simulink model "control_feedback_and_plant"  (R2023b)
settings: Solver=FixedStepAuto  StartTime=0.0  StopTime=500  FixedStep=0.01  RelTol=1e-3
settings Model: Creator=bhargavjha  LastModifiedBy=bhargavjha

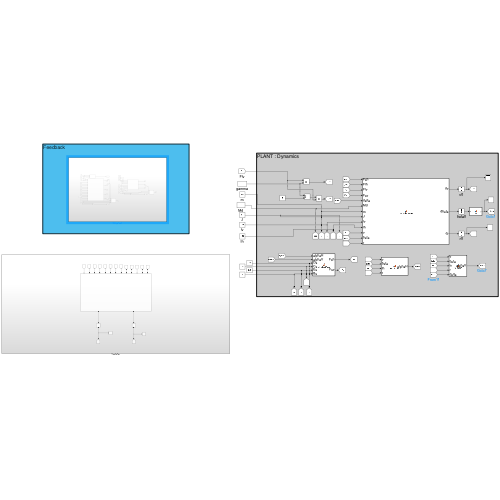
[thumbnail: Simulink's stored preview of the top-level diagram]
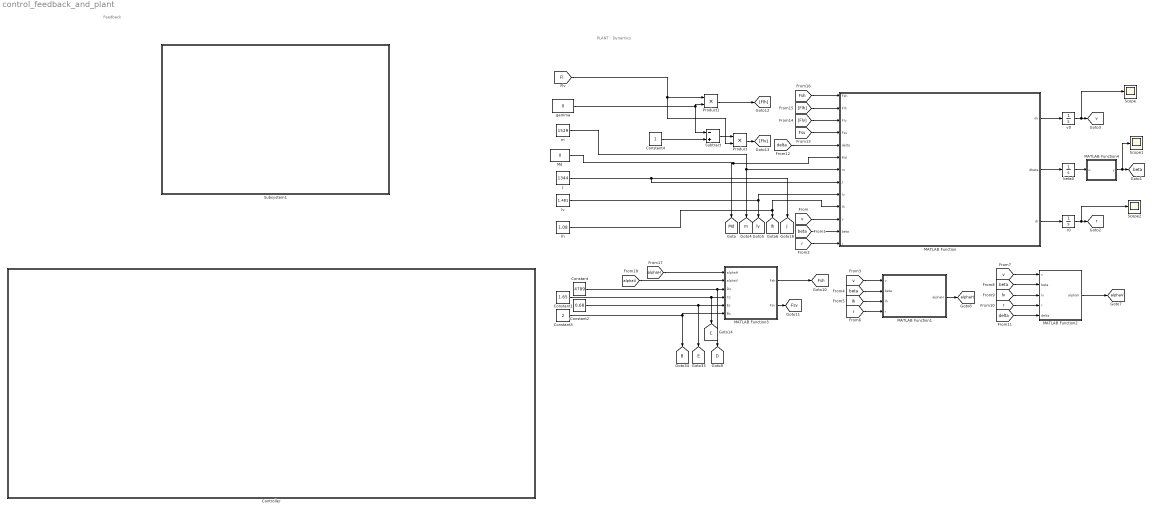
== system control_feedback_and_plant ==
  note: PLANT : Dynamics
  note: Feedback
  Constant : Constant  Value=4789
  Constant1 : Constant  Value=1.65
  Constant2 : Constant  Value=0.68
  Constant3 : Constant  Value=2
  Constant4 : Constant
  Controller : Subsystem
  J : Constant  Value=1344
  MATLAB Function : MATLAB Function  TreatAsAtomicUnit=on
  MATLAB Function1 : MATLAB Function  TreatAsAtomicUnit=on
  MATLAB Function2 : MATLAB Function  TreatAsAtomicUnit=on
  MATLAB Function3 : MATLAB Function  TreatAsAtomicUnit=on
  MATLAB Function4 : MATLAB Function  TreatAsAtomicUnit=on
  Md : Constant  Value=0
  Product : Product
  Product1 : Product
  Scope : Scope
  Scope1 : Scope
  Scope2 : Scope
  Subsystem1 : Subsystem
  Subtract : Sum  Inputs=-+
  beta0 : Integrator  InitialCondition=0.9
  gamma : Constant  Value=0
  lh : Constant  Value=1.08
  lv : Constant  Value=1.481
  m : Constant  Value=1529
  r0 : Integrator  InitialCondition=0.1
  v0 : Integrator  InitialCondition=0.1
  tag scope: B=global, C=global, D=global, E=global, Fsh=global, Fsv=global, J=global, Md=global, alphaH=global, alphaV=global, beta=global, lh=global, lv=global, m=global, r=global, v=global
  wires:
  [lv] -> MATLAB Function2/3(lv)
  MATLAB Function1/1(alphaH) -> [alphaH]
  MATLAB Function3/2(Fsv) -> [Fsv]
  v0/1 -> Scope/1, [v]
  lh/1 -> MATLAB Function/10(lh), [lh]
  MATLAB Function/1(dv) -> v0/1
  [beta] -> MATLAB Function1/2(beta)
  [v] -> MATLAB Function/11(v)
  J/1 -> [J], MATLAB Function/8(J)
  [Flh] -> MATLAB Function/2(Flh)
  Subtract/1 -> Product/1
  [Fsh] -> MATLAB Function/1(Fsh)
  m/1 -> [m], MATLAB Function/7(m)
  [v] -> MATLAB Function2/1(v)
  Product/1 -> [Flv]
  [r] -> MATLAB Function2/4(r)
  [v] -> MATLAB Function1/1(v)
  Constant3/1 -> MATLAB Function3/6(Bs), [B]
  gamma/1 -> Product1/2, Subtract/1
  lv/1 -> MATLAB Function/9(lv), [lv]
  [lh] -> MATLAB Function1/3(lh)
  MATLAB Function2/1(alphaV) -> [alphaV]
  Constant/1 -> [D], MATLAB Function3/3(Ds)
  Constant1/1 -> [C], MATLAB Function3/4(Cs)
  [beta] -> MATLAB Function/12(beta)
  Constant4/1 -> Subtract/2
  [delta] -> MATLAB Function/5(delta)
  Constant2/1 -> [E], MATLAB Function3/5(Es)
  MATLAB Function/3(dr) -> r0/1
  [alphaH] -> MATLAB Function3/1(alphaH)
  [Flv] -> MATLAB Function/3(Flv)
  [r] -> MATLAB Function/13(r)
  beta0/1 -> MATLAB Function4/1(u)
  MATLAB Function/2(dbeta) -> beta0/1
  [beta] -> MATLAB Function2/2(beta)
  Product1/1 -> [Flh]
  r0/1 -> Scope2/1, [r]
  [delta] -> MATLAB Function2/5(delta)
  [r] -> MATLAB Function1/4(r)
  MATLAB Function3/1(Fsh) -> [Fsh]
  Md/1 -> [Md], MATLAB Function/6(Md)
  [alphaV] -> MATLAB Function3/2(alphaV)
  [Fsv] -> MATLAB Function/4(Fsv)
  [Fl] -> Product/2, Product1/1
  MATLAB Function4/1(y) -> Scope1/1, [beta]

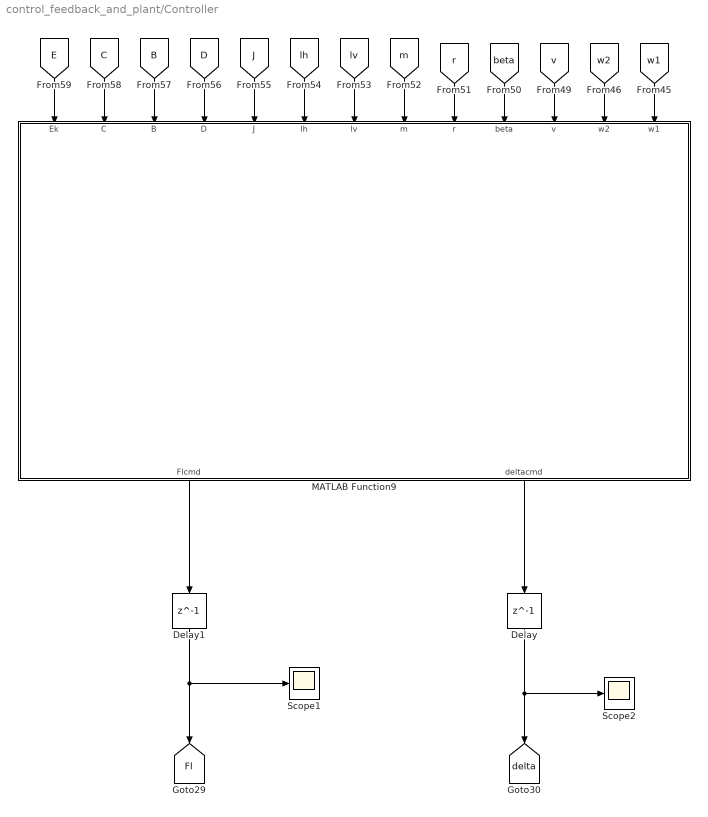
== system control_feedback_and_plant/Controller ==
  Delay : Delay  DelayLength=1
  Delay1 : Delay  DelayLength=1
  MATLAB Function9 : MATLAB Function  TreatAsAtomicUnit=on
  Scope1 : Scope
  Scope2 : Scope
  tag scope: Fl=global, delta=global
  wires:
  [B] -> MATLAB Function9/3(B)
  [C] -> MATLAB Function9/2(C)
  [E] -> MATLAB Function9/1(Ek)
  [lh] -> MATLAB Function9/6(lh)
  [w2] -> MATLAB Function9/12(w2)
  [m] -> MATLAB Function9/8(m)
  [beta] -> MATLAB Function9/10(beta)
  [w1] -> MATLAB Function9/13(w1)
  [D] -> MATLAB Function9/4(D)
  [J] -> MATLAB Function9/5(J)
  [r] -> MATLAB Function9/9(r)
  [lv] -> MATLAB Function9/7(lv)
  [v] -> MATLAB Function9/11(v)
  MATLAB Function9/2(deltacmd) -> Delay/1
  Delay/1 -> Scope2/1, [delta]
  Delay1/1 -> [Fl], Scope1/1
  MATLAB Function9/1(Flcmd) -> Delay1/1

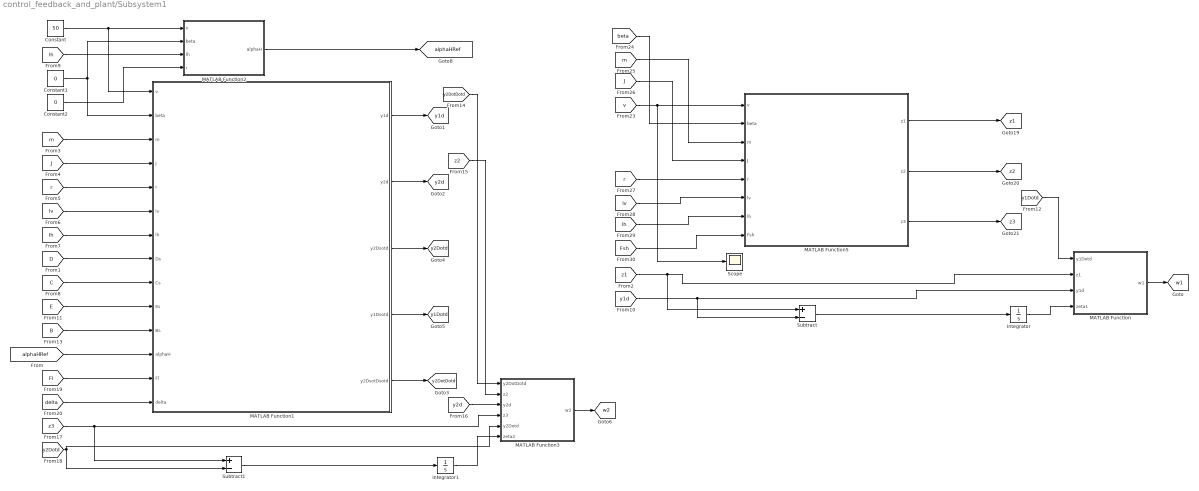
== system control_feedback_and_plant/Subsystem1 ==
  Constant : Constant  Value=50
  Constant1 : Constant  Value=0
  Constant2 : Constant  Value=0
  Integrator : Integrator
  Integrator1 : Integrator
  MATLAB Function : MATLAB Function  TreatAsAtomicUnit=on
  MATLAB Function1 : MATLAB Function  TreatAsAtomicUnit=on
  MATLAB Function2 : MATLAB Function  TreatAsAtomicUnit=on
  MATLAB Function3 : MATLAB Function  TreatAsAtomicUnit=on
  MATLAB Function5 : MATLAB Function  TreatAsAtomicUnit=on
  Scope : Scope
  Subtract : Sum  Inputs=+-
  Subtract1 : Sum  Inputs=+-
  tag scope: alphaHRef=global, w1=global, w2=global, y1Dotd=global, y1d=global, y2DotDotd=global, y2Dotd=global, y2d=global, z1=global, z2=global, z3=global
  wires:
  MATLAB Function3/1(w2) -> [w2]
  Integrator1/1 -> MATLAB Function3/6(zeta2)
  [y2d] -> MATLAB Function3/3(y2d)
  Integrator/1 -> MATLAB Function/4(zeta1)
  [y2DotDotd] -> MATLAB Function3/1(y2DotDotd)
  Subtract/1 -> Integrator/1
  Subtract1/1 -> Integrator1/1
  MATLAB Function1/5(y2DsotDsotd) -> [y2DotDotd]
  MATLAB Function1/4(y1Dsotd) -> [y1Dotd]
  MATLAB Function1/3(y2Dsotd) -> [y2Dotd]
  MATLAB Function1/2(y2d) -> [y2d]
  MATLAB Function2/1(alphaH) -> [alphaHRef]
  [z1] -> Subtract/1, MATLAB Function/2(z1)
  [Fsh] -> MATLAB Function5/8(Fsh)
  [lh] -> MATLAB Function5/7(lh)
  MATLAB Function/1(w1) -> [w1]
  [y1d] -> Subtract/2, MATLAB Function/3(y1d)
  [lv] -> MATLAB Function5/6(lv)
  [v] -> Scope/1, MATLAB Function5/1(v)
  MATLAB Function5/2(z2) -> [z2]
  [J] -> MATLAB Function5/4(J)
  [y1Dotd] -> MATLAB Function/1(y1Dotd)
  [z2] -> MATLAB Function3/2(z2)
  MATLAB Function5/1(z1) -> [z1]
  [m] -> MATLAB Function5/3(m)
  [beta] -> MATLAB Function5/2(beta)
  MATLAB Function5/3(z3) -> [z3]
  [r] -> MATLAB Function5/5(r)
  [lv] -> MATLAB Function1/6(lv)
  [delta] -> MATLAB Function1/14(delta)
  [alphaHRef] -> MATLAB Function1/12(alphaH)
  [B] -> MATLAB Function1/11(Bs)
  MATLAB Function1/1(y1d) -> [y1d]
  [z3] -> Subtract1/1, MATLAB Function3/4(z3)
  [E] -> MATLAB Function1/10(Es)
  [C] -> MATLAB Function1/9(Cs)
  [lh] -> MATLAB Function1/7(lh)
  [r] -> MATLAB Function1/5(r)
  [J] -> MATLAB Function1/4(J)
  Constant1/1 -> MATLAB Function1/2(beta), MATLAB Function2/2(beta)
  [y2Dotd] -> Subtract1/2, MATLAB Function3/5(y2Dotd)
  Constant2/1 -> MATLAB Function2/4(r)
  Constant/1 -> MATLAB Function2/1(v), MATLAB Function1/1(v)
  [Fl] -> MATLAB Function1/13(Fl)
  [lh] -> MATLAB Function2/3(lh)
  [D] -> MATLAB Function1/8(Ds)
  [m] -> MATLAB Function1/3(m)

== matlab function control_feedback_and_plant/Subsystem1/MATLAB Function5 ==
  data: v input; z1 output; beta input; m input; J input; r input; lv input; z2 output; lh input; Fsh input; z3 output
function [z1, z2, z3] = flatOutput_transform(v,beta,m,J,r,lv, lh, Fsh)

z1 = v*cos(beta);
z2 = v*sin(beta) - r*J/(m*lv);
z3 = ((lv+lh)/(m*lv))*Fsh - v*r*cos(beta);

== matlab function control_feedback_and_plant/Subsystem1/MATLAB Function2 ==
  data: v input; alphaH output; beta input; lh input; r input
function alphaH = cal_alphaH(v, beta, lh, r)

alphaH = -atan((v*sin(beta)-lh*r)/(v*cos(beta)));

== matlab function control_feedback_and_plant/MATLAB Function4 ==
  data: u input; y output
function y = fcn(u)
y=mod(mod(u,2*pi)+2*pi,2*pi);
%y = u;

== matlab function control_feedback_and_plant/Subsystem1/MATLAB Function ==
  data: y1Dotd input; w1 output; z1 input; y1d input; zeta1 input
function w1 = w1Calc(y1Dotd, z1,y1d,zeta1)

mu = 10;
mubar = 10;

w1 = y1Dotd-mu*(z1-y1d)-mubar*zeta1;

== matlab function control_feedback_and_plant/Controller/MATLAB Function9 ==
  data: Ek input; C input; B input; D input; J input; lh input; lv input; m input; r input; beta input; v input; w2 input; w1 input; Flcmd output; deltacmd output
function [Flcmd, deltacmd] = flatControl_To_RealControl(Ek, C, B, D, J, lh, lv, m, r, beta, v, w2, w1)



deltacmd=((-2).*B.*C.*D.*J.^(-1).*lv.*v.*cos(beta)+(-2).*B.^2.*C.^2.*D.^2.*...
  J.^(-1).*lv.^(-1).*(lh+lv).*m.^(-2).*(J+(-2).*lh.*lv.*m).*v.*cos ( ...
  beta).*(v.^2+cos(beta).^2.*(lh.*r+(-1).*v.*sin(beta)).^2).^(-1)+(-2).* ...
  B.^2.*C.^2.*D.^2.*lv.^(-1).*(lh+lv).*m.^(-2).*v.*cos(3.*beta).*(v.^2+ ...
  cos (beta).^2.*(lh.*r+(-1).*v.*sin(beta)).^2).^(-1)+(-4).*B.^2.*C.^2.* ...
  D.^2.*lh.*lv.^(-1).*(lh+lv).*m.^(-2).*r.*(v.^2+cos(beta).^2.*(lh.*r+( ...
  -1).*v.*sin(beta)).^2).^(-1).*sin(2.*beta)).^(-1).*(w2+2.*B.*C.*D.*J.^( ...
  -1).*lh.*v.*atan (cos(beta).*((-1).*lh.*r.*v.^(-1)+sin(beta))).*cos(beta)+( ...
  -2).*B.*C.*D.*J.^(-1).*lv.*v.*atan (cos(beta).*(lv.*r.*v.^(-1)+sin(beta)) ...
  ).*cos(beta)+r.*w1.*cos(beta).^2+(1/2).*r.^2.*v.*sin(beta)+(-1).*r.^2.*v.* ...
  cos (beta).^2.*sin(beta)+(1/2).*r.^2.*v.*cos(2.*beta).*sin(beta)+r.*w1.*sin(beta) ...
  .^2+(-1/2).*B.*C.*D.*lv.^(-1).*(lh+lv).*m.^(-1).*r.*v.^2.*(v.^2+ ...
  cos (beta).^2.*(lh.*r+(-1).*v.*sin(beta)).^2).^(-1)+(-1).*B.*C.*D.*lv.^( ...
  -1).*(lh+lv).*m.^(-1).*r.*(v.^2+(-2).*lh.*w1).*cos(2.*beta).*(v.^2+ ...
  cos (beta).^2.*(lh.*r+(-1).*v.*sin(beta)).^2).^(-1)+(-1/2).*B.*C.*D.* ...
  lv.^(-1).*(lh+lv).*m.^(-1).*r.*v.^2.*cos (4.*beta).*(v.^2+cos (beta).^2.*( ...
  lh.*r+(-1).*v.*sin(beta)).^2).^(-1)+(-1).*B.*C.*D.*lv.^(-1).*(lh+lv) ...
  .*m.^(-1).*v.*(lh.*r.^2+(-1).*w1).*sin (beta).*(v.^2+cos(beta).^2.*(lh.* ...
  r+(-1).*v.*sin(beta)).^2).^(-1)+(-4).*B.^2.*C.^2.*D.^2.*J.^(-1).*...
  lv.^(-1).*(lh+lv).*m.^(-2).*atan(cos(beta).*(lv.*r.*v.^(-1)+sin(beta))) ...
  .*cos (beta).*((-1).*lh.*lv.*m.*v+J.*v.*cos(2.*beta)+2.*J.*lh.*r.*sin(beta)) ...
  .*(v.^2+cos(beta).^2.*(lh.*r+(-1).*v.*sin(beta)).^2).^(-1)+(-4).*B.^2.* ...
  C.^2.*D.^2.*J.^(-1).*lv.^(-1).*(lh+lv).*m.^(-2).*atan (cos(beta).*(( ...
  -1).*lh.*r.*v.^(-1)+sin(beta))).*cos (beta).*(J.*v.*cos(2.*beta)+lh.*(lh.* ...
  m.*v+2.*J.*r.*sin(beta))).*(v.^2+cos(beta).^2.*(lh.*r+(-1).*v.*sin(beta)) ...
  .^2).^(-1)+(-1).*B.*C.*D.*lv.^(-1).*(lh+lv).*m.^(-1).*v.*(lh.* ...
  r.^2+w1).*(v.^2+cos(beta).^2.*(lh.*r+(-1).*v.*sin(beta)).^2).^(-1).*sin( ...
  3.*beta));



delta=mod(mod(deltacmd,2*pi)+2*pi,2*pi);
deltacmd = delta;

Flcmd=m.*w1+(-1).*m.*r.*v.*sin(beta)+2.*B.*C.*D.*delta.*sin(delta)+(-2).*B.*C.*D.* ...
  atan(cos(beta).*(lv.*r.*v.^(-1)+sin(beta))).*sin(delta);
delta;

== matlab function control_feedback_and_plant/Subsystem1/MATLAB Function3 ==
  data: y2DotDotd input; w2 output; z2 input; y2d input; z3 input; y2Dotd input; zeta2 input
function w2 = w2Calc(y2DotDotd,z2,y2d,z3,y2Dotd,zeta2)

nu1 = 1200;
nu2 = 60;
nubar = 8000;

w2 = y2DotDotd-nu1*(z2-y2d)-nu2*(z3-y2Dotd)-nubar*zeta2;

== matlab function control_feedback_and_plant/MATLAB Function1 ==
  data: v input; alphaH output; beta input; lh input; r input
function alphaH = cal_alphaH(v, beta, lh, r)

alphaH = -atan((v*sin(beta)-lh*r)/(v*cos(beta)));

== matlab function control_feedback_and_plant/MATLAB Function ==
  data: Fsh input; dv output; Flh input; Flv input; Fsv input; delta input; Md input; m input; J input; lv input; lh input; v input; beta input; r input; dbeta output; dr output
function [dv, dbeta, dr] = Car_Inner_Model(Fsh,Flh, Flv, Fsv, delta, Md, m, J, lv, lh, v, beta, r)


dv = (1/m)*(Fsv*sin(beta-delta)+Flv*cos(beta-delta)+Fsh*sin(beta)+Flh*cos(beta));

dbeta = -r + (1/(m*v))*(Fsv*cos(beta-delta)-Flv*sin(beta-delta)+Fsh*cos(beta)-Flh*sin(beta));

dr = (1/J)*(lv*(Fsv*cos(delta)+Flv*sin(delta))-lh*Fsh + Md);

end

== matlab function control_feedback_and_plant/MATLAB Function2 ==
  data: v input; alphaV output; beta input; lv input; r input; delta input
function alphaV = cal_alphaV(v, beta, lv, r, delta)

alphaV = delta-atan((v*sin(beta)+lv*r)/(v*cos(beta)));

== matlab function control_feedback_and_plant/MATLAB Function3 ==
  data: alphaH input; Fsh output; alphaV input; Fsv output; Ds input; Cs input; Es input; Bs input
function [Fsh, Fsv] = cal_lateralForce(alphaH, alphaV, Ds,Cs, Es, Bs)

%Es = 0;
Fsh = 2*Ds*(Cs*atan(Bs*alphaH));%sin(Cs*atan(Bs*alphaH-Es*(Bs*alphaH-atan(Bs*alphaH))));

Fsv = 2*Ds*(Cs*atan(Bs*alphaV));%sin(Cs*atan(Bs*alphaV-Es*(Bs*alphaV-atan(Bs*alphaV))));


%Fsv = 2*Ds*sin(Cs*atan(Bs*alphaV-Es*(Bs*alphaV-atan(Bs*alphaV))));


%Fsh = 2*Ds*sin(Cs*atan(Bs*alphaH-Es*(Bs*alphaH-atan(Bs*alphaH))));

== matlab function control_feedback_and_plant/Subsystem1/MATLAB Function1 ==
  data: v input; y1d output; y2d output; beta input; m input; J input; r input; lv input; y2Dsotd output; lh input; Ds input; Cs input; Es input; Bs input; alphaH input; y1Dsotd output; y2DsotDsotd output; Fl input; delta input
function [y1d, y2d, y2Dsotd, y1Dsotd, y2DsotDsotd] = flatOutput_transform(v,beta,m,J,r,lv, lh, Ds,Cs, Es, Bs, alphaH, Fl, delta)

%Fsh = 2*Ds*sin(Cs*atan(Bs*alphaH-Es*(Bs*alphaH-atan(Bs*alphaH))));
Fsh = 2*Ds*(Cs*(Bs*alphaH));

y1d = v*cos(beta);
y2d = v*sin(beta) - r*J/(m*lv);
y2Dsotd = ((lv+lh)/(m*lv))*Fsh - v*r*cos(beta);

 y1Dsotd =0; 
 %m.^(-1).*(Fl+m.*r.*v.*sin(beta)+2.*Bs.*Cs.*Ds.*((-1).*delta+atan(cos(beta).*( ...
%   lv.*r.*v.^(-1)+sin(beta)))).*sin(delta));

y2DsotDsotd = 0;
% (-2).*Bs.*Cs.*Ds.*J.^(-1).*v.*cos (beta).*(lh.*atan(cos(beta).*((-1).*lh.* ...
%   r.*v.^(-1)+sin(beta)))+lv.*(delta+(-1).*atan(cos(beta).*(lv.*r.*v.^(-1)+sin( ...
%   beta)))).*cos(delta))+(-1).*m.^(-1).*r.*sin(beta).*(m.*r.*v+2.*Bs.*Cs.*Ds.*( ...
%   atan (cos (beta).*((-1).*lh.*r.*v.^(-1)+sin(beta))).*cos(beta)+((-1).*delta+atan( ...
%   cos (beta).*(lv.*r.*v.^(-1)+sin(beta)))).*cos(beta+(-1).*delta))+Fl.*sin(beta))+ ...
%   m.^(-1).*r.*cos(beta).*((-1).*Fl.*cos(beta)+2.*Bs.*Cs.*Ds.*(atan (cos(beta).*(( ...
%   -1).*lh.*r.*v.^(-1)+sin(beta))).*sin(beta)+((-1).*delta+atan(cos (beta).*(lv.* ...
%   r.*v.^(-1)+sin(beta)))).*sin(beta+(-1).*delta)))+Bs.*Cs.*Ds.*J.^(-1).*lv.^(-1) ...
%   .*(lh+lv).*m.^(-2).*(v.^2+cos (beta).^2.*(lh.*r+(-1).*v.*sin(beta)).^2) ...
%   .^(-1).*(2.*J.*lh.*m.*r.^2.*v.*sin(beta)+(-4).*Bs.*Cs.*Ds.*(delta+(-1).* ...
%   atan(cos (beta).*(lv.*r.*v.^(-1)+sin(beta)))).*cos(beta).*cos (delta).*((-1).* ...
%   lh.*lv.*m.*v+J.*v.*cos(2.*beta)+2.*J.*lh.*r.*sin(beta))+2.*J.*cos(2.*beta) ...
%   .*((-1).*Fl.*lh.*r+m.*r.*v.^2+Fl.*v.*sin(beta))+4.*Bs.*Cs.*Ds.*atan(cos ( ...
%   beta).*((-1).*lh.*r.*v.^(-1)+sin(beta))).*cos(beta).*(J.*v.*cos(2.*beta)+lh.*( ...
%   lh.*m.*v+2.*J.*r.*sin(beta)))+4.*Bs.*Cs.*Ds.*J.*(delta+(-1).*atan(cos(beta).*( ...
%   lv.*r.*v.^(-1)+sin(beta)))).*cos(2.*beta).*(lh.*r+(-1).*v.*sin(beta)).*sin( ...
%   delta));
